simulink model "Intrgration"  (R2022b)
settings: Solver=VariableStepAuto  StartTime=0.0  StopTime=10.0  RelTol=1e-3
libraries: simulink x1
settings Model: Creator=LYZ  LastModifiedBy=LYZ

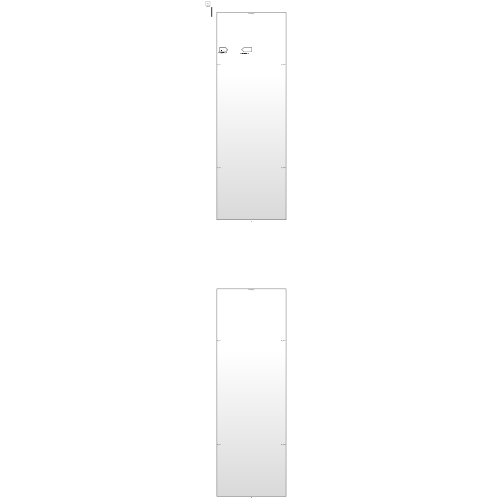
[thumbnail: Simulink's stored preview of the top-level diagram]
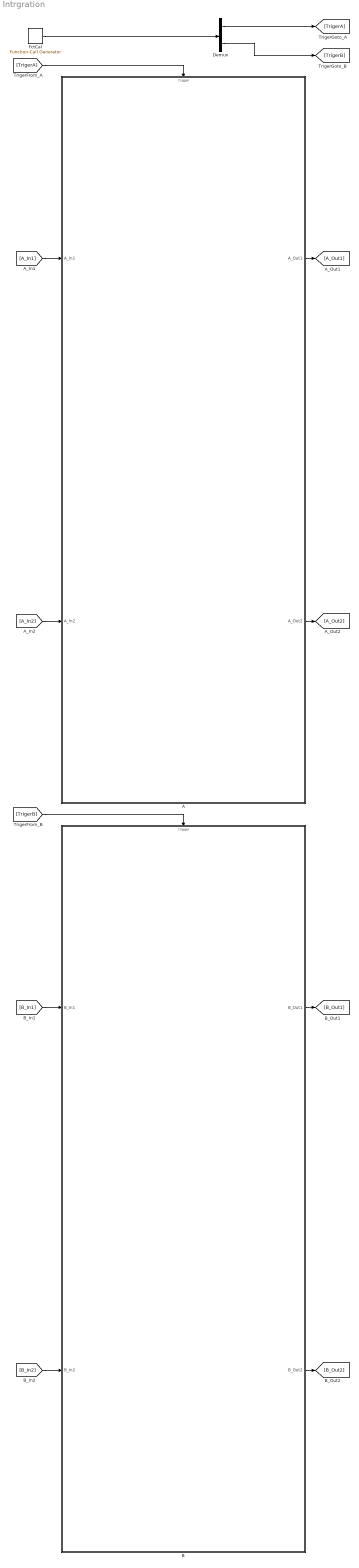
== system Intrgration ==
  A : Subsystem
  B : Subsystem
  Demux : Demux  Outputs=2
  FctCal : simulink/Ports & Subsystems/Function-Call Generator  sample_time=1  numberOfIterations=1  DisallowWideOutput=off
  wires:
  A/1(A_Out1) -> [A_Out1]
  FctCal/1 -> Demux/1
  [TrigerA] -> A/Trigger
  [B_In1] -> B/1(B_In1)
  [TrigerB] -> B/Trigger
  [A_In1] -> A/1(A_In1)
  [B_In2] -> B/2(B_In2)
  [A_In2] -> A/2(A_In2)
  Demux/1 -> [TrigerA]
  A/2(A_Out2) -> [A_Out2]
  Demux/2 -> [TrigerB]
  B/1(B_Out1) -> [B_Out1]
  B/2(B_Out2) -> [B_Out2]

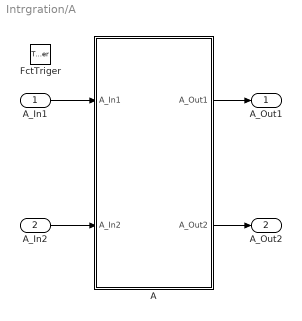
== system Intrgration/A ==
  A_In1 : Inport
  A_In2 : Inport  Port=2
  FctTriger : TriggerPort  TriggerType=function-call  VariantControl=(inherit)  PortDimensions=1
  A : Subsystem
  A_Out1 : Outport
  A_Out2 : Outport  Port=2
  wires:
  A_In1/1 -> A/1(A_In1)
  A_In2/1 -> A/2(A_In2)
  A/2(A_Out2) -> A_Out2/1
  A/1(A_Out1) -> A_Out1/1

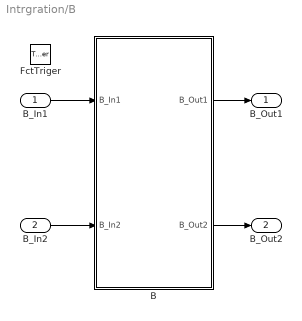
== system Intrgration/B ==
  B_In1 : Inport
  B_In2 : Inport  Port=2
  FctTriger : TriggerPort  TriggerType=function-call  VariantControl=(inherit)  PortDimensions=1
  B : Subsystem
  B_Out1 : Outport
  B_Out2 : Outport  Port=2
  wires:
  B_In1/1 -> B/1(B_In1)
  B_In2/1 -> B/2(B_In2)
  B/1(B_Out1) -> B_Out1/1
  B/2(B_Out2) -> B_Out2/1

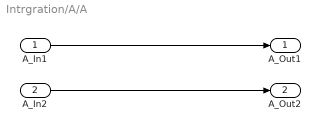
== system Intrgration/A/A ==
  A_In1 : Inport
  A_In2 : Inport  Port=2
  A_Out1 : Outport
  A_Out2 : Outport  Port=2
  wires:
  A_In2/1 -> A_Out2/1
  A_In1/1 -> A_Out1/1

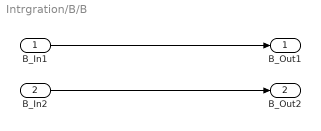
== system Intrgration/B/B ==
  B_In1 : Inport
  B_In2 : Inport  Port=2
  B_Out1 : Outport
  B_Out2 : Outport  Port=2
  wires:
  B_In2/1 -> B_Out2/1
  B_In1/1 -> B_Out1/1
